simulink model "PreBraking_Scenario2_cs"  (R2014b)
settings: Solver=ode5  SolverMode=SingleTasking  StartTime=0.0  StopTime=inf  FixedStep=1/100  RelTol=1e-3
PreLoadFcn:
  | mbxruntime.callbacks.PreLoadFcn(bdroot);
  | check_NUTS_defined;
  | 
  | assignin('base',['model_closed_' bdroot],false);addpath('../includes_AEBS');
PostLoadFcn:
  | mbxruntime.callbacks.PostLoadFcn(bdroot);
InitFcn:
  | mbxruntime.callbacks.InitFcn(bdroot);
StartFcn:
  | mbxruntime.callbacks.StartFcn(bdroot);
StopFcn:
  | mbxruntime.callbacks.StopFcn(bdroot);
model workspace: external: MAT-File .\PreBraking_Scenario2_cs_hws.mat (data not in the file)
undefined symbols (not defined in the file or in its folder): mbxruntime, OrientationPitch, OrientationRoll, PositionX, PositionY, PositionZ, tabledata, warningInitialVelocity, x0
undefined symbols (not defined in the file): PreBraking_Scenario2_cs_03ca8bbbeab2b9b9, PreBraking_Scenario2_cs_060f8d532884bc4b, PreBraking_Scenario2_cs_06c37d8c8719462d, PreBraking_Scenario2_cs_0d3de4e10595602b, PreBraking_Scenario2_cs_132afc293d4bc970, PreBraking_Scenario2_cs_135fb3525bf57813, PreBraking_Scenario2_cs_199db523920b0ae8, PreBraking_Scenario2_cs_19b5c7fc995ca371, PreBraking_Scenario2_cs_1c0d05c0e95fb3bc, PreBraking_Scenario2_cs_230ed70c3742a1eb, PreBraking_Scenario2_cs_2a9a795ed7b4eca0, PreBraking_Scenario2_cs_2aad3e26cef81116, PreBraking_Scenario2_cs_3112792458948f16, PreBraking_Scenario2_cs_31511e5cf664957f, PreBraking_Scenario2_cs_335bc07f9f9d6bb2, PreBraking_Scenario2_cs_343e102d67d9e47c, PreBraking_Scenario2_cs_38754ff77a13247b, PreBraking_Scenario2_cs_3f42c52076d9af39, PreBraking_Scenario2_cs_4b3e07bd10cdcbdf, PreBraking_Scenario2_cs_4d97be448e41c5e7, PreBraking_Scenario2_cs_50fbc7e9b9a11bbd, PreBraking_Scenario2_cs_54739860340bd271, PreBraking_Scenario2_cs_5a356ab1c62c8f7e, PreBraking_Scenario2_cs_5b4437f6719e0d1b, PreBraking_Scenario2_cs_5c234b912a76c6a5, PreBraking_Scenario2_cs_6168355cd5f7aa5b, PreBraking_Scenario2_cs_622a303a40218b4d, PreBraking_Scenario2_cs_647713569694f0a8, PreBraking_Scenario2_cs_69cfdaef90de11b6, PreBraking_Scenario2_cs_6af59d93ed31b258, PreBraking_Scenario2_cs_6b0b2c155afad700, PreBraking_Scenario2_cs_6b0e277e7fb709ae, PreBraking_Scenario2_cs_6cdb8944f433c9b5, PreBraking_Scenario2_cs_6e61e0d6d53946a8, PreBraking_Scenario2_cs_721bd4ea87d705e5, PreBraking_Scenario2_cs_733181add4a3a2bd, PreBraking_Scenario2_cs_7a4dfa61d77329b3, PreBraking_Scenario2_cs_7b6eba6e821515af, PreBraking_Scenario2_cs_7dfcf0aa2939e252, PreBraking_Scenario2_cs_7f39d304a27b340b, PreBraking_Scenario2_cs_8077b8dca741d53f, PreBraking_Scenario2_cs_83874eeccd6bc572, PreBraking_Scenario2_cs_8e3f6b53dcde3bb3, PreBraking_Scenario2_cs_98c5cdaae36d0717, PreBraking_Scenario2_cs_98cfc98f5f5b01fc, PreBraking_Scenario2_cs_9906f28f708d2a62, PreBraking_Scenario2_cs_a13988e047af266f, PreBraking_Scenario2_cs_a8fd4bfaed66c690, PreBraking_Scenario2_cs_a93f6bf774ad8002, PreBraking_Scenario2_cs_a9ad9a9d247ad05d, PreBraking_Scenario2_cs_ab408108b3f0fc97, PreBraking_Scenario2_cs_Audi_A8_3_Dynamics_Simple_initialPitch, PreBraking_Scenario2_cs_Audi_A8_3_Dynamics_Simple_initialRoll, PreBraking_Scenario2_cs_Audi_A8_3_Dynamics_Simple_initialX, PreBraking_Scenario2_cs_Audi_A8_3_Dynamics_Simple_initialY, PreBraking_Scenario2_cs_Audi_A8_3_Dynamics_Simple_initialYaw, PreBraking_Scenario2_cs_Audi_A8_3_Dynamics_Simple_initialZ, PreBraking_Scenario2_cs_b1fc7fed98e6f1a7, PreBraking_Scenario2_cs_b75ef87da1419b4e, PreBraking_Scenario2_cs_b7a6524fab202de5 ... (+41)
libraries: simulink_extras x81, PreScanSimulinkLibrary x27, simulink x20, PreScanUsefulBlocks x2
(part 23 of 33)

== system PreBraking_Scenario2_cs/VISUMatrixSign_HighwayOverhang_2/Actuator ==
  VISUMatrixSign_HighwayOverhang_2 : Inport  Tag=inport/VisuMatrixSign  SampleTime=1/100  BusOutputAsStruct=on
  DemuxVisuMatrixSign : Demux
  visu_MatrixSign_13 : S-Function  FunctionName=sfun_ResourceNameSelector  Parameters=mbxruntime.parameters.convert(UniqueID), mbxruntime.parameters.convert(ResourceList), mbxruntime.parameters.convert(PivotName),tabledata, TimeStep  EnableBusSupport=off  mask(PreScan Sink Block: VisuMatrixSign){UniqueID=394, ResourceList={'2' 'InformationSign\stop.jpg' '3' 'InformationSign\MatrixSign_GreenArrow.png' '4' 'InformationSign\MatrixSign_Speed_50.png' }, PivotName=/child:name=MatrixSign_13/trafficSignElement, TimeStep=1/100}
      mask prompts: UniqueID "Parent Unique Identifier (auto-generated)"; ResourceList "Resource List (auto-generated)"; PivotName "Name of pivot (auto-generated)"; TimeStep "Simulink time step"
      mask help:
      | The VisuMatrixSign block provides a way to adapt the texture of the plates connected to an overhang, based on Resource IDs of the texture files.
      |
      | For more information, please click Help.
      mask init:
      | [tabledata] = mbxruntime.parameters.table(UniqueID,ResourceList,PivotName);
      mask Help: eval('openHelp(733)')
      mask Display: image(imread('HighwaySpeedMatrix.png'))
  visu_MatrixSign_14 : S-Function  FunctionName=sfun_ResourceNameSelector  Parameters=mbxruntime.parameters.convert(UniqueID), mbxruntime.parameters.convert(ResourceList), mbxruntime.parameters.convert(PivotName),tabledata, TimeStep  EnableBusSupport=off  mask(PreScan Sink Block: VisuMatrixSign){UniqueID=394, ResourceList={'2' 'InformationSign\stop.jpg' '3' 'InformationSign\MatrixSign_GreenArrow.png' '4' 'InformationSign\MatrixSign_Speed_50.png' }, PivotName=/child:name=MatrixSign_14/trafficSignElement, TimeStep=1/100}
      mask prompts: UniqueID "Parent Unique Identifier (auto-generated)"; ResourceList "Resource List (auto-generated)"; PivotName "Name of pivot (auto-generated)"; TimeStep "Simulink time step"
      mask help:
      | The VisuMatrixSign block provides a way to adapt the texture of the plates connected to an overhang, based on Resource IDs of the texture files.
      |
      | For more information, please click Help.
      mask init:
      | [tabledata] = mbxruntime.parameters.table(UniqueID,ResourceList,PivotName);
      mask Help: eval('openHelp(733)')
      mask Display: image(imread('HighwaySpeedMatrix.png'))
  visu_MatrixSign_15 : S-Function  FunctionName=sfun_ResourceNameSelector  Parameters=mbxruntime.parameters.convert(UniqueID), mbxruntime.parameters.convert(ResourceList), mbxruntime.parameters.convert(PivotName),tabledata, TimeStep  EnableBusSupport=off  mask(PreScan Sink Block: VisuMatrixSign){UniqueID=394, ResourceList={'2' 'InformationSign\stop.jpg' '3' 'InformationSign\MatrixSign_GreenArrow.png' '4' 'InformationSign\MatrixSign_Speed_50.png' }, PivotName=/child:name=MatrixSign_15/trafficSignElement, TimeStep=1/100}
      mask prompts: UniqueID "Parent Unique Identifier (auto-generated)"; ResourceList "Resource List (auto-generated)"; PivotName "Name of pivot (auto-generated)"; TimeStep "Simulink time step"
      mask help:
      | The VisuMatrixSign block provides a way to adapt the texture of the plates connected to an overhang, based on Resource IDs of the texture files.
      |
      | For more information, please click Help.
      mask init:
      | [tabledata] = mbxruntime.parameters.table(UniqueID,ResourceList,PivotName);
      mask Help: eval('openHelp(733)')
      mask Display: image(imread('HighwaySpeedMatrix.png'))
  visu_MatrixSign_16 : S-Function  FunctionName=sfun_ResourceNameSelector  Parameters=mbxruntime.parameters.convert(UniqueID), mbxruntime.parameters.convert(ResourceList), mbxruntime.parameters.convert(PivotName),tabledata, TimeStep  EnableBusSupport=off  mask(PreScan Sink Block: VisuMatrixSign){UniqueID=394, ResourceList={'2' 'InformationSign\stop.jpg' '3' 'InformationSign\MatrixSign_GreenArrow.png' '4' 'InformationSign\MatrixSign_Speed_50.png' }, PivotName=/child:name=MatrixSign_16/trafficSignElement, TimeStep=1/100}
      mask prompts: UniqueID "Parent Unique Identifier (auto-generated)"; ResourceList "Resource List (auto-generated)"; PivotName "Name of pivot (auto-generated)"; TimeStep "Simulink time step"
      mask help:
      | The VisuMatrixSign block provides a way to adapt the texture of the plates connected to an overhang, based on Resource IDs of the texture files.
      |
      | For more information, please click Help.
      mask init:
      | [tabledata] = mbxruntime.parameters.table(UniqueID,ResourceList,PivotName);
      mask Help: eval('openHelp(733)')
      mask Display: image(imread('HighwaySpeedMatrix.png'))
  wires:
  VISUMatrixSign_HighwayOverhang_2/1 -> DemuxVisuMatrixSign/1
  DemuxVisuMatrixSign/1 -> visu_MatrixSign_13/1
  DemuxVisuMatrixSign/2 -> visu_MatrixSign_14/1
  DemuxVisuMatrixSign/3 -> visu_MatrixSign_15/1
  DemuxVisuMatrixSign/4 -> visu_MatrixSign_16/1

== system PreBraking_Scenario2_cs/VISUMatrixSign_HighwayOverhang_3/Actuator ==
  VISUMatrixSign_HighwayOverhang_3 : Inport  Tag=inport/VisuMatrixSign  SampleTime=1/100  BusOutputAsStruct=on
  DemuxVisuMatrixSign : Demux
  visu_MatrixSign_5 : S-Function  FunctionName=sfun_ResourceNameSelector  Parameters=mbxruntime.parameters.convert(UniqueID), mbxruntime.parameters.convert(ResourceList), mbxruntime.parameters.convert(PivotName),tabledata, TimeStep  EnableBusSupport=off  mask(PreScan Sink Block: VisuMatrixSign){UniqueID=395, ResourceList={'2' 'InformationSign\stop.jpg' '3' 'InformationSign\MatrixSign_GreenArrow.png' '4' 'InformationSign\MatrixSign_Speed_50.png' }, PivotName=/child:name=MatrixSign_5/trafficSignElement, TimeStep=1/100}
      mask prompts: UniqueID "Parent Unique Identifier (auto-generated)"; ResourceList "Resource List (auto-generated)"; PivotName "Name of pivot (auto-generated)"; TimeStep "Simulink time step"
      mask help:
      | The VisuMatrixSign block provides a way to adapt the texture of the plates connected to an overhang, based on Resource IDs of the texture files.
      |
      | For more information, please click Help.
      mask init:
      | [tabledata] = mbxruntime.parameters.table(UniqueID,ResourceList,PivotName);
      mask Help: eval('openHelp(733)')
      mask Display: image(imread('HighwaySpeedMatrix.png'))
  visu_MatrixSign_6 : S-Function  FunctionName=sfun_ResourceNameSelector  Parameters=mbxruntime.parameters.convert(UniqueID), mbxruntime.parameters.convert(ResourceList), mbxruntime.parameters.convert(PivotName),tabledata, TimeStep  EnableBusSupport=off  mask(PreScan Sink Block: VisuMatrixSign){UniqueID=395, ResourceList={'2' 'InformationSign\stop.jpg' '3' 'InformationSign\MatrixSign_GreenArrow.png' '4' 'InformationSign\MatrixSign_Speed_50.png' }, PivotName=/child:name=MatrixSign_6/trafficSignElement, TimeStep=1/100}
      mask prompts: UniqueID "Parent Unique Identifier (auto-generated)"; ResourceList "Resource List (auto-generated)"; PivotName "Name of pivot (auto-generated)"; TimeStep "Simulink time step"
      mask help:
      | The VisuMatrixSign block provides a way to adapt the texture of the plates connected to an overhang, based on Resource IDs of the texture files.
      |
      | For more information, please click Help.
      mask init:
      | [tabledata] = mbxruntime.parameters.table(UniqueID,ResourceList,PivotName);
      mask Help: eval('openHelp(733)')
      mask Display: image(imread('HighwaySpeedMatrix.png'))
  visu_MatrixSign_7 : S-Function  FunctionName=sfun_ResourceNameSelector  Parameters=mbxruntime.parameters.convert(UniqueID), mbxruntime.parameters.convert(ResourceList), mbxruntime.parameters.convert(PivotName),tabledata, TimeStep  EnableBusSupport=off  mask(PreScan Sink Block: VisuMatrixSign){UniqueID=395, ResourceList={'2' 'InformationSign\stop.jpg' '3' 'InformationSign\MatrixSign_GreenArrow.png' '4' 'InformationSign\MatrixSign_Speed_50.png' }, PivotName=/child:name=MatrixSign_7/trafficSignElement, TimeStep=1/100}
      mask prompts: UniqueID "Parent Unique Identifier (auto-generated)"; ResourceList "Resource List (auto-generated)"; PivotName "Name of pivot (auto-generated)"; TimeStep "Simulink time step"
      mask help:
      | The VisuMatrixSign block provides a way to adapt the texture of the plates connected to an overhang, based on Resource IDs of the texture files.
      |
      | For more information, please click Help.
      mask init:
      | [tabledata] = mbxruntime.parameters.table(UniqueID,ResourceList,PivotName);
      mask Help: eval('openHelp(733)')
      mask Display: image(imread('HighwaySpeedMatrix.png'))
  visu_MatrixSign_8 : S-Function  FunctionName=sfun_ResourceNameSelector  Parameters=mbxruntime.parameters.convert(UniqueID), mbxruntime.parameters.convert(ResourceList), mbxruntime.parameters.convert(PivotName),tabledata, TimeStep  EnableBusSupport=off  mask(PreScan Sink Block: VisuMatrixSign){UniqueID=395, ResourceList={'2' 'InformationSign\stop.jpg' '3' 'InformationSign\MatrixSign_GreenArrow.png' '4' 'InformationSign\MatrixSign_Speed_50.png' }, PivotName=/child:name=MatrixSign_8/trafficSignElement, TimeStep=1/100}
      mask prompts: UniqueID "Parent Unique Identifier (auto-generated)"; ResourceList "Resource List (auto-generated)"; PivotName "Name of pivot (auto-generated)"; TimeStep "Simulink time step"
      mask help:
      | The VisuMatrixSign block provides a way to adapt the texture of the plates connected to an overhang, based on Resource IDs of the texture files.
      |
      | For more information, please click Help.
      mask init:
      | [tabledata] = mbxruntime.parameters.table(UniqueID,ResourceList,PivotName);
      mask Help: eval('openHelp(733)')
      mask Display: image(imread('HighwaySpeedMatrix.png'))
  wires:
  VISUMatrixSign_HighwayOverhang_3/1 -> DemuxVisuMatrixSign/1
  DemuxVisuMatrixSign/1 -> visu_MatrixSign_5/1
  DemuxVisuMatrixSign/2 -> visu_MatrixSign_6/1
  DemuxVisuMatrixSign/3 -> visu_MatrixSign_7/1
  DemuxVisuMatrixSign/4 -> visu_MatrixSign_8/1

== system PreBraking_Scenario2_cs/VISUMatrixSign_HighwayOverhang_4/Actuator ==
  VISUMatrixSign_HighwayOverhang_4 : Inport  Tag=inport/VisuMatrixSign  SampleTime=1/100  BusOutputAsStruct=on
  DemuxVisuMatrixSign : Demux
  visu_MatrixSign_10 : S-Function  FunctionName=sfun_ResourceNameSelector  Parameters=mbxruntime.parameters.convert(UniqueID), mbxruntime.parameters.convert(ResourceList), mbxruntime.parameters.convert(PivotName),tabledata, TimeStep  EnableBusSupport=off  mask(PreScan Sink Block: VisuMatrixSign){UniqueID=396, ResourceList={'2' 'InformationSign\stop.jpg' '3' 'InformationSign\MatrixSign_GreenArrow.png' '4' 'InformationSign\MatrixSign_Speed_50.png' }, PivotName=/child:name=MatrixSign_10/trafficSignElement, TimeStep=1/100}
      mask prompts: UniqueID "Parent Unique Identifier (auto-generated)"; ResourceList "Resource List (auto-generated)"; PivotName "Name of pivot (auto-generated)"; TimeStep "Simulink time step"
      mask help:
      | The VisuMatrixSign block provides a way to adapt the texture of the plates connected to an overhang, based on Resource IDs of the texture files.
      |
      | For more information, please click Help.
      mask init:
      | [tabledata] = mbxruntime.parameters.table(UniqueID,ResourceList,PivotName);
      mask Help: eval('openHelp(733)')
      mask Display: image(imread('HighwaySpeedMatrix.png'))
  visu_MatrixSign_11 : S-Function  FunctionName=sfun_ResourceNameSelector  Parameters=mbxruntime.parameters.convert(UniqueID), mbxruntime.parameters.convert(ResourceList), mbxruntime.parameters.convert(PivotName),tabledata, TimeStep  EnableBusSupport=off  mask(PreScan Sink Block: VisuMatrixSign){UniqueID=396, ResourceList={'2' 'InformationSign\stop.jpg' '3' 'InformationSign\MatrixSign_GreenArrow.png' '4' 'InformationSign\MatrixSign_Speed_50.png' }, PivotName=/child:name=MatrixSign_11/trafficSignElement, TimeStep=1/100}
      mask prompts: UniqueID "Parent Unique Identifier (auto-generated)"; ResourceList "Resource List (auto-generated)"; PivotName "Name of pivot (auto-generated)"; TimeStep "Simulink time step"
      mask help:
      | The VisuMatrixSign block provides a way to adapt the texture of the plates connected to an overhang, based on Resource IDs of the texture files.
      |
      | For more information, please click Help.
      mask init:
      | [tabledata] = mbxruntime.parameters.table(UniqueID,ResourceList,PivotName);
      mask Help: eval('openHelp(733)')
      mask Display: image(imread('HighwaySpeedMatrix.png'))
  visu_MatrixSign_12 : S-Function  FunctionName=sfun_ResourceNameSelector  Parameters=mbxruntime.parameters.convert(UniqueID), mbxruntime.parameters.convert(ResourceList), mbxruntime.parameters.convert(PivotName),tabledata, TimeStep  EnableBusSupport=off  mask(PreScan Sink Block: VisuMatrixSign){UniqueID=396, ResourceList={'2' 'InformationSign\stop.jpg' '3' 'InformationSign\MatrixSign_GreenArrow.png' '4' 'InformationSign\MatrixSign_Speed_50.png' }, PivotName=/child:name=MatrixSign_12/trafficSignElement, TimeStep=1/100}
      mask prompts: UniqueID "Parent Unique Identifier (auto-generated)"; ResourceList "Resource List (auto-generated)"; PivotName "Name of pivot (auto-generated)"; TimeStep "Simulink time step"
      mask help:
      | The VisuMatrixSign block provides a way to adapt the texture of the plates connected to an overhang, based on Resource IDs of the texture files.
      |
      | For more information, please click Help.
      mask init:
      | [tabledata] = mbxruntime.parameters.table(UniqueID,ResourceList,PivotName);
      mask Help: eval('openHelp(733)')
      mask Display: image(imread('HighwaySpeedMatrix.png'))
  visu_MatrixSign_9 : S-Function  FunctionName=sfun_ResourceNameSelector  Parameters=mbxruntime.parameters.convert(UniqueID), mbxruntime.parameters.convert(ResourceList), mbxruntime.parameters.convert(PivotName),tabledata, TimeStep  EnableBusSupport=off  mask(PreScan Sink Block: VisuMatrixSign){UniqueID=396, ResourceList={'2' 'InformationSign\stop.jpg' '3' 'InformationSign\MatrixSign_GreenArrow.png' '4' 'InformationSign\MatrixSign_Speed_50.png' }, PivotName=/child:name=MatrixSign_9/trafficSignElement, TimeStep=1/100}
      mask prompts: UniqueID "Parent Unique Identifier (auto-generated)"; ResourceList "Resource List (auto-generated)"; PivotName "Name of pivot (auto-generated)"; TimeStep "Simulink time step"
      mask help:
      | The VisuMatrixSign block provides a way to adapt the texture of the plates connected to an overhang, based on Resource IDs of the texture files.
      |
      | For more information, please click Help.
      mask init:
      | [tabledata] = mbxruntime.parameters.table(UniqueID,ResourceList,PivotName);
      mask Help: eval('openHelp(733)')
      mask Display: image(imread('HighwaySpeedMatrix.png'))
  wires:
  VISUMatrixSign_HighwayOverhang_4/1 -> DemuxVisuMatrixSign/1
  DemuxVisuMatrixSign/1 -> visu_MatrixSign_9/1
  DemuxVisuMatrixSign/2 -> visu_MatrixSign_10/1
  DemuxVisuMatrixSign/3 -> visu_MatrixSign_11/1
  DemuxVisuMatrixSign/4 -> visu_MatrixSign_12/1

== system PreBraking_Scenario2_cs/WheelL0_Audi_A8_3/Actuator ==
  Joint : Inport
  Bus Selector : BusSelector  OutputSignals=POSITION,ORIENTATION
  visu_Rotate : Subsystem  mask(RPYActuator){UniqueID=UniqueID, Object3DID=Rotate_ObjectID3D, TimeStep=TimeStep}
      mask prompts: UniqueID "Auto-Assigned: Unique ID"; Object3DID "Auto-Assigned: Child 3D Object ID"; TimeStep "Auto-Assigned: Upload Period [s]"
      mask help: Applies angles update to selected child object
      mask Help:
      | Applies position update to selected child object
      | 
      | - UniqueID (double)   : Unique ID of the parent actor
      | - Object3DID (string) : Name of the child 3D object
      mask Display: port_label('input', 1, ['visu_Rotate_' Object3DID])
  visu_Translate : Subsystem  mask(PositionActuator){UniqueID=UniqueID, Object3DID=Translate_ObjectID3D, TimeStep=TimeStep}
      mask prompts: UniqueID "Auto-Assigned: Unique ID"; Object3DID "Auto-Assigned: Child 3D Object ID"; TimeStep "Auto-Assigned: Upload Period [s]"
      mask help: Applies position update to selected child object
      mask Help:
      | Applies position update to selected child object
      | 
      | - UniqueID (double)   : Unique ID of the parent actor
      | - Object3DID (string) : Name of the child 3D object
      mask Display: port_label('input', 1, ['visu_Translate_' Object3DID])
  wires:
  Bus Selector/2 -> visu_Rotate/1(In1)  "<ORIENTATION>"
  Bus Selector/1 -> visu_Translate/1(In1)  "<POSITION>"
  Joint/1 -> Bus Selector/1

== system PreBraking_Scenario2_cs/WheelL0_BMW_X5_2/Actuator ==
  Joint : Inport
  Bus Selector : BusSelector  OutputSignals=POSITION,ORIENTATION
  visu_Rotate : Subsystem  mask(RPYActuator){UniqueID=UniqueID, Object3DID=Rotate_ObjectID3D, TimeStep=TimeStep}
      mask prompts: UniqueID "Auto-Assigned: Unique ID"; Object3DID "Auto-Assigned: Child 3D Object ID"; TimeStep "Auto-Assigned: Upload Period [s]"
      mask help: Applies angles update to selected child object
      mask Help:
      | Applies position update to selected child object
      | 
      | - UniqueID (double)   : Unique ID of the parent actor
      | - Object3DID (string) : Name of the child 3D object
      mask Display: port_label('input', 1, ['visu_Rotate_' Object3DID])
  visu_Translate : Subsystem  mask(PositionActuator){UniqueID=UniqueID, Object3DID=Translate_ObjectID3D, TimeStep=TimeStep}
      mask prompts: UniqueID "Auto-Assigned: Unique ID"; Object3DID "Auto-Assigned: Child 3D Object ID"; TimeStep "Auto-Assigned: Upload Period [s]"
      mask help: Applies position update to selected child object
      mask Help:
      | Applies position update to selected child object
      | 
      | - UniqueID (double)   : Unique ID of the parent actor
      | - Object3DID (string) : Name of the child 3D object
      mask Display: port_label('input', 1, ['visu_Translate_' Object3DID])
  wires:
  Bus Selector/2 -> visu_Rotate/1(In1)  "<ORIENTATION>"
  Bus Selector/1 -> visu_Translate/1(In1)  "<POSITION>"
  Joint/1 -> Bus Selector/1

== system PreBraking_Scenario2_cs/WheelL0_BMW_X5_3/Actuator ==
  Joint : Inport
  Bus Selector : BusSelector  OutputSignals=POSITION,ORIENTATION
  visu_Rotate : Subsystem  mask(RPYActuator){UniqueID=UniqueID, Object3DID=Rotate_ObjectID3D, TimeStep=TimeStep}
      mask prompts: UniqueID "Auto-Assigned: Unique ID"; Object3DID "Auto-Assigned: Child 3D Object ID"; TimeStep "Auto-Assigned: Upload Period [s]"
      mask help: Applies angles update to selected child object
      mask Help:
      | Applies position update to selected child object
      | 
      | - UniqueID (double)   : Unique ID of the parent actor
      | - Object3DID (string) : Name of the child 3D object
      mask Display: port_label('input', 1, ['visu_Rotate_' Object3DID])
  visu_Translate : Subsystem  mask(PositionActuator){UniqueID=UniqueID, Object3DID=Translate_ObjectID3D, TimeStep=TimeStep}
      mask prompts: UniqueID "Auto-Assigned: Unique ID"; Object3DID "Auto-Assigned: Child 3D Object ID"; TimeStep "Auto-Assigned: Upload Period [s]"
      mask help: Applies position update to selected child object
      mask Help:
      | Applies position update to selected child object
      | 
      | - UniqueID (double)   : Unique ID of the parent actor
      | - Object3DID (string) : Name of the child 3D object
      mask Display: port_label('input', 1, ['visu_Translate_' Object3DID])
  wires:
  Bus Selector/2 -> visu_Rotate/1(In1)  "<ORIENTATION>"
  Bus Selector/1 -> visu_Translate/1(In1)  "<POSITION>"
  Joint/1 -> Bus Selector/1

== system PreBraking_Scenario2_cs/WheelL0_BMW_Z3_2/Actuator ==
  Joint : Inport
  Bus Selector : BusSelector  OutputSignals=POSITION,ORIENTATION
  visu_Rotate : Subsystem  mask(RPYActuator){UniqueID=UniqueID, Object3DID=Rotate_ObjectID3D, TimeStep=TimeStep}
      mask prompts: UniqueID "Auto-Assigned: Unique ID"; Object3DID "Auto-Assigned: Child 3D Object ID"; TimeStep "Auto-Assigned: Upload Period [s]"
      mask help: Applies angles update to selected child object
      mask Help:
      | Applies position update to selected child object
      | 
      | - UniqueID (double)   : Unique ID of the parent actor
      | - Object3DID (string) : Name of the child 3D object
      mask Display: port_label('input', 1, ['visu_Rotate_' Object3DID])
  visu_Translate : Subsystem  mask(PositionActuator){UniqueID=UniqueID, Object3DID=Translate_ObjectID3D, TimeStep=TimeStep}
      mask prompts: UniqueID "Auto-Assigned: Unique ID"; Object3DID "Auto-Assigned: Child 3D Object ID"; TimeStep "Auto-Assigned: Upload Period [s]"
      mask help: Applies position update to selected child object
      mask Help:
      | Applies position update to selected child object
      | 
      | - UniqueID (double)   : Unique ID of the parent actor
      | - Object3DID (string) : Name of the child 3D object
      mask Display: port_label('input', 1, ['visu_Translate_' Object3DID])
  wires:
  Bus Selector/2 -> visu_Rotate/1(In1)  "<ORIENTATION>"
  Bus Selector/1 -> visu_Translate/1(In1)  "<POSITION>"
  Joint/1 -> Bus Selector/1

== system PreBraking_Scenario2_cs/WheelL0_Citroen_C3_2/Actuator ==
  Joint : Inport
  Bus Selector : BusSelector  OutputSignals=POSITION,ORIENTATION
  visu_Rotate : Subsystem  mask(RPYActuator){UniqueID=UniqueID, Object3DID=Rotate_ObjectID3D, TimeStep=TimeStep}
      mask prompts: UniqueID "Auto-Assigned: Unique ID"; Object3DID "Auto-Assigned: Child 3D Object ID"; TimeStep "Auto-Assigned: Upload Period [s]"
      mask help: Applies angles update to selected child object
      mask Help:
      | Applies position update to selected child object
      | 
      | - UniqueID (double)   : Unique ID of the parent actor
      | - Object3DID (string) : Name of the child 3D object
      mask Display: port_label('input', 1, ['visu_Rotate_' Object3DID])
  visu_Translate : Subsystem  mask(PositionActuator){UniqueID=UniqueID, Object3DID=Translate_ObjectID3D, TimeStep=TimeStep}
      mask prompts: UniqueID "Auto-Assigned: Unique ID"; Object3DID "Auto-Assigned: Child 3D Object ID"; TimeStep "Auto-Assigned: Upload Period [s]"
      mask help: Applies position update to selected child object
      mask Help:
      | Applies position update to selected child object
      | 
      | - UniqueID (double)   : Unique ID of the parent actor
      | - Object3DID (string) : Name of the child 3D object
      mask Display: port_label('input', 1, ['visu_Translate_' Object3DID])
  wires:
  Bus Selector/2 -> visu_Rotate/1(In1)  "<ORIENTATION>"
  Bus Selector/1 -> visu_Translate/1(In1)  "<POSITION>"
  Joint/1 -> Bus Selector/1

== system PreBraking_Scenario2_cs/WheelL0_Fiat_Bravo_2/Actuator ==
  Joint : Inport
  Bus Selector : BusSelector  OutputSignals=POSITION,ORIENTATION
  visu_Rotate : Subsystem  mask(RPYActuator){UniqueID=UniqueID, Object3DID=Rotate_ObjectID3D, TimeStep=TimeStep}
      mask prompts: UniqueID "Auto-Assigned: Unique ID"; Object3DID "Auto-Assigned: Child 3D Object ID"; TimeStep "Auto-Assigned: Upload Period [s]"
      mask help: Applies angles update to selected child object
      mask Help:
      | Applies position update to selected child object
      | 
      | - UniqueID (double)   : Unique ID of the parent actor
      | - Object3DID (string) : Name of the child 3D object
      mask Display: port_label('input', 1, ['visu_Rotate_' Object3DID])
  visu_Translate : Subsystem  mask(PositionActuator){UniqueID=UniqueID, Object3DID=Translate_ObjectID3D, TimeStep=TimeStep}
      mask prompts: UniqueID "Auto-Assigned: Unique ID"; Object3DID "Auto-Assigned: Child 3D Object ID"; TimeStep "Auto-Assigned: Upload Period [s]"
      mask help: Applies position update to selected child object
      mask Help:
      | Applies position update to selected child object
      | 
      | - UniqueID (double)   : Unique ID of the parent actor
      | - Object3DID (string) : Name of the child 3D object
      mask Display: port_label('input', 1, ['visu_Translate_' Object3DID])
  wires:
  Bus Selector/2 -> visu_Rotate/1(In1)  "<ORIENTATION>"
  Bus Selector/1 -> visu_Translate/1(In1)  "<POSITION>"
  Joint/1 -> Bus Selector/1

== system PreBraking_Scenario2_cs/WheelL0_Ford_Fiesta_2/Actuator ==
  Joint : Inport
  Bus Selector : BusSelector  OutputSignals=POSITION,ORIENTATION
  visu_Rotate : Subsystem  mask(RPYActuator){UniqueID=UniqueID, Object3DID=Rotate_ObjectID3D, TimeStep=TimeStep}
      mask prompts: UniqueID "Auto-Assigned: Unique ID"; Object3DID "Auto-Assigned: Child 3D Object ID"; TimeStep "Auto-Assigned: Upload Period [s]"
      mask help: Applies angles update to selected child object
      mask Help:
      | Applies position update to selected child object
      | 
      | - UniqueID (double)   : Unique ID of the parent actor
      | - Object3DID (string) : Name of the child 3D object
      mask Display: port_label('input', 1, ['visu_Rotate_' Object3DID])
  visu_Translate : Subsystem  mask(PositionActuator){UniqueID=UniqueID, Object3DID=Translate_ObjectID3D, TimeStep=TimeStep}
      mask prompts: UniqueID "Auto-Assigned: Unique ID"; Object3DID "Auto-Assigned: Child 3D Object ID"; TimeStep "Auto-Assigned: Upload Period [s]"
      mask help: Applies position update to selected child object
      mask Help:
      | Applies position update to selected child object
      | 
      | - UniqueID (double)   : Unique ID of the parent actor
      | - Object3DID (string) : Name of the child 3D object
      mask Display: port_label('input', 1, ['visu_Translate_' Object3DID])
  wires:
  Bus Selector/2 -> visu_Rotate/1(In1)  "<ORIENTATION>"
  Bus Selector/1 -> visu_Translate/1(In1)  "<POSITION>"
  Joint/1 -> Bus Selector/1

== system PreBraking_Scenario2_cs/WheelL0_Toyota_Previa_2/Actuator ==
  Joint : Inport
  Bus Selector : BusSelector  OutputSignals=POSITION,ORIENTATION
  visu_Rotate : Subsystem  mask(RPYActuator){UniqueID=UniqueID, Object3DID=Rotate_ObjectID3D, TimeStep=TimeStep}
      mask prompts: UniqueID "Auto-Assigned: Unique ID"; Object3DID "Auto-Assigned: Child 3D Object ID"; TimeStep "Auto-Assigned: Upload Period [s]"
      mask help: Applies angles update to selected child object
      mask Help:
      | Applies position update to selected child object
      | 
      | - UniqueID (double)   : Unique ID of the parent actor
      | - Object3DID (string) : Name of the child 3D object
      mask Display: port_label('input', 1, ['visu_Rotate_' Object3DID])
  visu_Translate : Subsystem  mask(PositionActuator){UniqueID=UniqueID, Object3DID=Translate_ObjectID3D, TimeStep=TimeStep}
      mask prompts: UniqueID "Auto-Assigned: Unique ID"; Object3DID "Auto-Assigned: Child 3D Object ID"; TimeStep "Auto-Assigned: Upload Period [s]"
      mask help: Applies position update to selected child object
      mask Help:
      | Applies position update to selected child object
      | 
      | - UniqueID (double)   : Unique ID of the parent actor
      | - Object3DID (string) : Name of the child 3D object
      mask Display: port_label('input', 1, ['visu_Translate_' Object3DID])
  wires:
  Bus Selector/2 -> visu_Rotate/1(In1)  "<ORIENTATION>"
  Bus Selector/1 -> visu_Translate/1(In1)  "<POSITION>"
  Joint/1 -> Bus Selector/1

== system PreBraking_Scenario2_cs/WheelL0_Toyota_Previa_3/Actuator ==
  Joint : Inport
  Bus Selector : BusSelector  OutputSignals=POSITION,ORIENTATION
  visu_Rotate : Subsystem  mask(RPYActuator){UniqueID=UniqueID, Object3DID=Rotate_ObjectID3D, TimeStep=TimeStep}
      mask prompts: UniqueID "Auto-Assigned: Unique ID"; Object3DID "Auto-Assigned: Child 3D Object ID"; TimeStep "Auto-Assigned: Upload Period [s]"
      mask help: Applies angles update to selected child object
      mask Help:
      | Applies position update to selected child object
      | 
      | - UniqueID (double)   : Unique ID of the parent actor
      | - Object3DID (string) : Name of the child 3D object
      mask Display: port_label('input', 1, ['visu_Rotate_' Object3DID])
  visu_Translate : Subsystem  mask(PositionActuator){UniqueID=UniqueID, Object3DID=Translate_ObjectID3D, TimeStep=TimeStep}
      mask prompts: UniqueID "Auto-Assigned: Unique ID"; Object3DID "Auto-Assigned: Child 3D Object ID"; TimeStep "Auto-Assigned: Upload Period [s]"
      mask help: Applies position update to selected child object
      mask Help:
      | Applies position update to selected child object
      | 
      | - UniqueID (double)   : Unique ID of the parent actor
      | - Object3DID (string) : Name of the child 3D object
      mask Display: port_label('input', 1, ['visu_Translate_' Object3DID])
  wires:
  Bus Selector/2 -> visu_Rotate/1(In1)  "<ORIENTATION>"
  Bus Selector/1 -> visu_Translate/1(In1)  "<POSITION>"
  Joint/1 -> Bus Selector/1

== system PreBraking_Scenario2_cs/WheelL1_Audi_A8_3/Actuator ==
  Joint : Inport
  Bus Selector : BusSelector  OutputSignals=POSITION,ORIENTATION
  visu_Rotate : Subsystem  mask(RPYActuator){UniqueID=UniqueID, Object3DID=Rotate_ObjectID3D, TimeStep=TimeStep}
      mask prompts: UniqueID "Auto-Assigned: Unique ID"; Object3DID "Auto-Assigned: Child 3D Object ID"; TimeStep "Auto-Assigned: Upload Period [s]"
      mask help: Applies angles update to selected child object
      mask Help:
      | Applies position update to selected child object
      | 
      | - UniqueID (double)   : Unique ID of the parent actor
      | - Object3DID (string) : Name of the child 3D object
      mask Display: port_label('input', 1, ['visu_Rotate_' Object3DID])
  visu_Translate : Subsystem  mask(PositionActuator){UniqueID=UniqueID, Object3DID=Translate_ObjectID3D, TimeStep=TimeStep}
      mask prompts: UniqueID "Auto-Assigned: Unique ID"; Object3DID "Auto-Assigned: Child 3D Object ID"; TimeStep "Auto-Assigned: Upload Period [s]"
      mask help: Applies position update to selected child object
      mask Help:
      | Applies position update to selected child object
      | 
      | - UniqueID (double)   : Unique ID of the parent actor
      | - Object3DID (string) : Name of the child 3D object
      mask Display: port_label('input', 1, ['visu_Translate_' Object3DID])
  wires:
  Bus Selector/2 -> visu_Rotate/1(In1)  "<ORIENTATION>"
  Bus Selector/1 -> visu_Translate/1(In1)  "<POSITION>"
  Joint/1 -> Bus Selector/1

== system PreBraking_Scenario2_cs/WheelL1_BMW_X5_2/Actuator ==
  Joint : Inport
  Bus Selector : BusSelector  OutputSignals=POSITION,ORIENTATION
  visu_Rotate : Subsystem  mask(RPYActuator){UniqueID=UniqueID, Object3DID=Rotate_ObjectID3D, TimeStep=TimeStep}
      mask prompts: UniqueID "Auto-Assigned: Unique ID"; Object3DID "Auto-Assigned: Child 3D Object ID"; TimeStep "Auto-Assigned: Upload Period [s]"
      mask help: Applies angles update to selected child object
      mask Help:
      | Applies position update to selected child object
      | 
      | - UniqueID (double)   : Unique ID of the parent actor
      | - Object3DID (string) : Name of the child 3D object
      mask Display: port_label('input', 1, ['visu_Rotate_' Object3DID])
  visu_Translate : Subsystem  mask(PositionActuator){UniqueID=UniqueID, Object3DID=Translate_ObjectID3D, TimeStep=TimeStep}
      mask prompts: UniqueID "Auto-Assigned: Unique ID"; Object3DID "Auto-Assigned: Child 3D Object ID"; TimeStep "Auto-Assigned: Upload Period [s]"
      mask help: Applies position update to selected child object
      mask Help:
      | Applies position update to selected child object
      | 
      | - UniqueID (double)   : Unique ID of the parent actor
      | - Object3DID (string) : Name of the child 3D object
      mask Display: port_label('input', 1, ['visu_Translate_' Object3DID])
  wires:
  Bus Selector/2 -> visu_Rotate/1(In1)  "<ORIENTATION>"
  Bus Selector/1 -> visu_Translate/1(In1)  "<POSITION>"
  Joint/1 -> Bus Selector/1

== system PreBraking_Scenario2_cs/WheelL1_BMW_X5_3/Actuator ==
  Joint : Inport
  Bus Selector : BusSelector  OutputSignals=POSITION,ORIENTATION
  visu_Rotate : Subsystem  mask(RPYActuator){UniqueID=UniqueID, Object3DID=Rotate_ObjectID3D, TimeStep=TimeStep}
      mask prompts: UniqueID "Auto-Assigned: Unique ID"; Object3DID "Auto-Assigned: Child 3D Object ID"; TimeStep "Auto-Assigned: Upload Period [s]"
      mask help: Applies angles update to selected child object
      mask Help:
      | Applies position update to selected child object
      | 
      | - UniqueID (double)   : Unique ID of the parent actor
      | - Object3DID (string) : Name of the child 3D object
      mask Display: port_label('input', 1, ['visu_Rotate_' Object3DID])
  visu_Translate : Subsystem  mask(PositionActuator){UniqueID=UniqueID, Object3DID=Translate_ObjectID3D, TimeStep=TimeStep}
      mask prompts: UniqueID "Auto-Assigned: Unique ID"; Object3DID "Auto-Assigned: Child 3D Object ID"; TimeStep "Auto-Assigned: Upload Period [s]"
      mask help: Applies position update to selected child object
      mask Help:
      | Applies position update to selected child object
      | 
      | - UniqueID (double)   : Unique ID of the parent actor
      | - Object3DID (string) : Name of the child 3D object
      mask Display: port_label('input', 1, ['visu_Translate_' Object3DID])
  wires:
  Bus Selector/2 -> visu_Rotate/1(In1)  "<ORIENTATION>"
  Bus Selector/1 -> visu_Translate/1(In1)  "<POSITION>"
  Joint/1 -> Bus Selector/1

== system PreBraking_Scenario2_cs/WheelL1_BMW_Z3_2/Actuator ==
  Joint : Inport
  Bus Selector : BusSelector  OutputSignals=POSITION,ORIENTATION
  visu_Rotate : Subsystem  mask(RPYActuator){UniqueID=UniqueID, Object3DID=Rotate_ObjectID3D, TimeStep=TimeStep}
      mask prompts: UniqueID "Auto-Assigned: Unique ID"; Object3DID "Auto-Assigned: Child 3D Object ID"; TimeStep "Auto-Assigned: Upload Period [s]"
      mask help: Applies angles update to selected child object
      mask Help:
      | Applies position update to selected child object
      | 
      | - UniqueID (double)   : Unique ID of the parent actor
      | - Object3DID (string) : Name of the child 3D object
      mask Display: port_label('input', 1, ['visu_Rotate_' Object3DID])
  visu_Translate : Subsystem  mask(PositionActuator){UniqueID=UniqueID, Object3DID=Translate_ObjectID3D, TimeStep=TimeStep}
      mask prompts: UniqueID "Auto-Assigned: Unique ID"; Object3DID "Auto-Assigned: Child 3D Object ID"; TimeStep "Auto-Assigned: Upload Period [s]"
      mask help: Applies position update to selected child object
      mask Help:
      | Applies position update to selected child object
      | 
      | - UniqueID (double)   : Unique ID of the parent actor
      | - Object3DID (string) : Name of the child 3D object
      mask Display: port_label('input', 1, ['visu_Translate_' Object3DID])
  wires:
  Bus Selector/2 -> visu_Rotate/1(In1)  "<ORIENTATION>"
  Bus Selector/1 -> visu_Translate/1(In1)  "<POSITION>"
  Joint/1 -> Bus Selector/1

== system PreBraking_Scenario2_cs/WheelL1_Citroen_C3_2/Actuator ==
  Joint : Inport
  Bus Selector : BusSelector  OutputSignals=POSITION,ORIENTATION
  visu_Rotate : Subsystem  mask(RPYActuator){UniqueID=UniqueID, Object3DID=Rotate_ObjectID3D, TimeStep=TimeStep}
      mask prompts: UniqueID "Auto-Assigned: Unique ID"; Object3DID "Auto-Assigned: Child 3D Object ID"; TimeStep "Auto-Assigned: Upload Period [s]"
      mask help: Applies angles update to selected child object
      mask Help:
      | Applies position update to selected child object
      | 
      | - UniqueID (double)   : Unique ID of the parent actor
      | - Object3DID (string) : Name of the child 3D object
      mask Display: port_label('input', 1, ['visu_Rotate_' Object3DID])
  visu_Translate : Subsystem  mask(PositionActuator){UniqueID=UniqueID, Object3DID=Translate_ObjectID3D, TimeStep=TimeStep}
      mask prompts: UniqueID "Auto-Assigned: Unique ID"; Object3DID "Auto-Assigned: Child 3D Object ID"; TimeStep "Auto-Assigned: Upload Period [s]"
      mask help: Applies position update to selected child object
      mask Help:
      | Applies position update to selected child object
      | 
      | - UniqueID (double)   : Unique ID of the parent actor
      | - Object3DID (string) : Name of the child 3D object
      mask Display: port_label('input', 1, ['visu_Translate_' Object3DID])
  wires:
  Bus Selector/2 -> visu_Rotate/1(In1)  "<ORIENTATION>"
  Bus Selector/1 -> visu_Translate/1(In1)  "<POSITION>"
  Joint/1 -> Bus Selector/1

== system PreBraking_Scenario2_cs/WheelL1_Fiat_Bravo_2/Actuator ==
  Joint : Inport
  Bus Selector : BusSelector  OutputSignals=POSITION,ORIENTATION
  visu_Rotate : Subsystem  mask(RPYActuator){UniqueID=UniqueID, Object3DID=Rotate_ObjectID3D, TimeStep=TimeStep}
      mask prompts: UniqueID "Auto-Assigned: Unique ID"; Object3DID "Auto-Assigned: Child 3D Object ID"; TimeStep "Auto-Assigned: Upload Period [s]"
      mask help: Applies angles update to selected child object
      mask Help:
      | Applies position update to selected child object
      | 
      | - UniqueID (double)   : Unique ID of the parent actor
      | - Object3DID (string) : Name of the child 3D object
      mask Display: port_label('input', 1, ['visu_Rotate_' Object3DID])
  visu_Translate : Subsystem  mask(PositionActuator){UniqueID=UniqueID, Object3DID=Translate_ObjectID3D, TimeStep=TimeStep}
      mask prompts: UniqueID "Auto-Assigned: Unique ID"; Object3DID "Auto-Assigned: Child 3D Object ID"; TimeStep "Auto-Assigned: Upload Period [s]"
      mask help: Applies position update to selected child object
      mask Help:
      | Applies position update to selected child object
      | 
      | - UniqueID (double)   : Unique ID of the parent actor
      | - Object3DID (string) : Name of the child 3D object
      mask Display: port_label('input', 1, ['visu_Translate_' Object3DID])
  wires:
  Bus Selector/2 -> visu_Rotate/1(In1)  "<ORIENTATION>"
  Bus Selector/1 -> visu_Translate/1(In1)  "<POSITION>"
  Joint/1 -> Bus Selector/1

== system PreBraking_Scenario2_cs/WheelL1_Ford_Fiesta_2/Actuator ==
  Joint : Inport
  Bus Selector : BusSelector  OutputSignals=POSITION,ORIENTATION
  visu_Rotate : Subsystem  mask(RPYActuator){UniqueID=UniqueID, Object3DID=Rotate_ObjectID3D, TimeStep=TimeStep}
      mask prompts: UniqueID "Auto-Assigned: Unique ID"; Object3DID "Auto-Assigned: Child 3D Object ID"; TimeStep "Auto-Assigned: Upload Period [s]"
      mask help: Applies angles update to selected child object
      mask Help:
      | Applies position update to selected child object
      | 
      | - UniqueID (double)   : Unique ID of the parent actor
      | - Object3DID (string) : Name of the child 3D object
      mask Display: port_label('input', 1, ['visu_Rotate_' Object3DID])
  visu_Translate : Subsystem  mask(PositionActuator){UniqueID=UniqueID, Object3DID=Translate_ObjectID3D, TimeStep=TimeStep}
      mask prompts: UniqueID "Auto-Assigned: Unique ID"; Object3DID "Auto-Assigned: Child 3D Object ID"; TimeStep "Auto-Assigned: Upload Period [s]"
      mask help: Applies position update to selected child object
      mask Help:
      | Applies position update to selected child object
      | 
      | - UniqueID (double)   : Unique ID of the parent actor
      | - Object3DID (string) : Name of the child 3D object
      mask Display: port_label('input', 1, ['visu_Translate_' Object3DID])
  wires:
  Bus Selector/2 -> visu_Rotate/1(In1)  "<ORIENTATION>"
  Bus Selector/1 -> visu_Translate/1(In1)  "<POSITION>"
  Joint/1 -> Bus Selector/1

== system PreBraking_Scenario2_cs/WheelL1_Toyota_Previa_2/Actuator ==
  Joint : Inport
  Bus Selector : BusSelector  OutputSignals=POSITION,ORIENTATION
  visu_Rotate : Subsystem  mask(RPYActuator){UniqueID=UniqueID, Object3DID=Rotate_ObjectID3D, TimeStep=TimeStep}
      mask prompts: UniqueID "Auto-Assigned: Unique ID"; Object3DID "Auto-Assigned: Child 3D Object ID"; TimeStep "Auto-Assigned: Upload Period [s]"
      mask help: Applies angles update to selected child object
      mask Help:
      | Applies position update to selected child object
      | 
      | - UniqueID (double)   : Unique ID of the parent actor
      | - Object3DID (string) : Name of the child 3D object
      mask Display: port_label('input', 1, ['visu_Rotate_' Object3DID])
  visu_Translate : Subsystem  mask(PositionActuator){UniqueID=UniqueID, Object3DID=Translate_ObjectID3D, TimeStep=TimeStep}
      mask prompts: UniqueID "Auto-Assigned: Unique ID"; Object3DID "Auto-Assigned: Child 3D Object ID"; TimeStep "Auto-Assigned: Upload Period [s]"
      mask help: Applies position update to selected child object
      mask Help:
      | Applies position update to selected child object
      | 
      | - UniqueID (double)   : Unique ID of the parent actor
      | - Object3DID (string) : Name of the child 3D object
      mask Display: port_label('input', 1, ['visu_Translate_' Object3DID])
  wires:
  Bus Selector/2 -> visu_Rotate/1(In1)  "<ORIENTATION>"
  Bus Selector/1 -> visu_Translate/1(In1)  "<POSITION>"
  Joint/1 -> Bus Selector/1

== system PreBraking_Scenario2_cs/WheelL1_Toyota_Previa_3/Actuator ==
  Joint : Inport
  Bus Selector : BusSelector  OutputSignals=POSITION,ORIENTATION
  visu_Rotate : Subsystem  mask(RPYActuator){UniqueID=UniqueID, Object3DID=Rotate_ObjectID3D, TimeStep=TimeStep}
      mask prompts: UniqueID "Auto-Assigned: Unique ID"; Object3DID "Auto-Assigned: Child 3D Object ID"; TimeStep "Auto-Assigned: Upload Period [s]"
      mask help: Applies angles update to selected child object
      mask Help:
      | Applies position update to selected child object
      | 
      | - UniqueID (double)   : Unique ID of the parent actor
      | - Object3DID (string) : Name of the child 3D object
      mask Display: port_label('input', 1, ['visu_Rotate_' Object3DID])
  visu_Translate : Subsystem  mask(PositionActuator){UniqueID=UniqueID, Object3DID=Translate_ObjectID3D, TimeStep=TimeStep}
      mask prompts: UniqueID "Auto-Assigned: Unique ID"; Object3DID "Auto-Assigned: Child 3D Object ID"; TimeStep "Auto-Assigned: Upload Period [s]"
      mask help: Applies position update to selected child object
      mask Help:
      | Applies position update to selected child object
      | 
      | - UniqueID (double)   : Unique ID of the parent actor
      | - Object3DID (string) : Name of the child 3D object
      mask Display: port_label('input', 1, ['visu_Translate_' Object3DID])
  wires:
  Bus Selector/2 -> visu_Rotate/1(In1)  "<ORIENTATION>"
  Bus Selector/1 -> visu_Translate/1(In1)  "<POSITION>"
  Joint/1 -> Bus Selector/1

== system PreBraking_Scenario2_cs/WheelR0_Audi_A8_3/Actuator ==
  Joint : Inport
  Bus Selector : BusSelector  OutputSignals=POSITION,ORIENTATION
  visu_Rotate : Subsystem  mask(RPYActuator){UniqueID=UniqueID, Object3DID=Rotate_ObjectID3D, TimeStep=TimeStep}
      mask prompts: UniqueID "Auto-Assigned: Unique ID"; Object3DID "Auto-Assigned: Child 3D Object ID"; TimeStep "Auto-Assigned: Upload Period [s]"
      mask help: Applies angles update to selected child object
      mask Help:
      | Applies position update to selected child object
      | 
      | - UniqueID (double)   : Unique ID of the parent actor
      | - Object3DID (string) : Name of the child 3D object
      mask Display: port_label('input', 1, ['visu_Rotate_' Object3DID])
  visu_Translate : Subsystem  mask(PositionActuator){UniqueID=UniqueID, Object3DID=Translate_ObjectID3D, TimeStep=TimeStep}
      mask prompts: UniqueID "Auto-Assigned: Unique ID"; Object3DID "Auto-Assigned: Child 3D Object ID"; TimeStep "Auto-Assigned: Upload Period [s]"
      mask help: Applies position update to selected child object
      mask Help:
      | Applies position update to selected child object
      | 
      | - UniqueID (double)   : Unique ID of the parent actor
      | - Object3DID (string) : Name of the child 3D object
      mask Display: port_label('input', 1, ['visu_Translate_' Object3DID])
  wires:
  Bus Selector/2 -> visu_Rotate/1(In1)  "<ORIENTATION>"
  Bus Selector/1 -> visu_Translate/1(In1)  "<POSITION>"
  Joint/1 -> Bus Selector/1

== system PreBraking_Scenario2_cs/WheelR0_BMW_X5_2/Actuator ==
  Joint : Inport
  Bus Selector : BusSelector  OutputSignals=POSITION,ORIENTATION
  visu_Rotate : Subsystem  mask(RPYActuator){UniqueID=UniqueID, Object3DID=Rotate_ObjectID3D, TimeStep=TimeStep}
      mask prompts: UniqueID "Auto-Assigned: Unique ID"; Object3DID "Auto-Assigned: Child 3D Object ID"; TimeStep "Auto-Assigned: Upload Period [s]"
      mask help: Applies angles update to selected child object
      mask Help:
      | Applies position update to selected child object
      | 
      | - UniqueID (double)   : Unique ID of the parent actor
      | - Object3DID (string) : Name of the child 3D object
      mask Display: port_label('input', 1, ['visu_Rotate_' Object3DID])
  visu_Translate : Subsystem  mask(PositionActuator){UniqueID=UniqueID, Object3DID=Translate_ObjectID3D, TimeStep=TimeStep}
      mask prompts: UniqueID "Auto-Assigned: Unique ID"; Object3DID "Auto-Assigned: Child 3D Object ID"; TimeStep "Auto-Assigned: Upload Period [s]"
      mask help: Applies position update to selected child object
      mask Help:
      | Applies position update to selected child object
      | 
      | - UniqueID (double)   : Unique ID of the parent actor
      | - Object3DID (string) : Name of the child 3D object
      mask Display: port_label('input', 1, ['visu_Translate_' Object3DID])
  wires:
  Bus Selector/2 -> visu_Rotate/1(In1)  "<ORIENTATION>"
  Bus Selector/1 -> visu_Translate/1(In1)  "<POSITION>"
  Joint/1 -> Bus Selector/1
